simulink model "Fig264"  (R2014b)
settings: Solver=FixedStepDiscrete  StartTime=0.0  StopTime=.2  RelTol=1e-3
libraries: dspsigops x1
settings Model: Creator=Dennis Silage  LastModifiedBy=Silage
settings DataIOCC: SignalLoggingSaveFormat=ModelDataLogs
settings OptimizationCC: ExpressionDepthLimit=2147483647  InitFltsAndDblsToZero=on
settings DebuggingCC: UnderspecifiedInitializationDetection=Classic  MergeDetectMultiDrivingBlocksExec=none  FcnCallInpInsideContextMsg=UseLocalSettings  StateNameClashWarn=warning
settings GRTTargetCC: CombineOutputUpdateFcns=off  GRTInterface=on

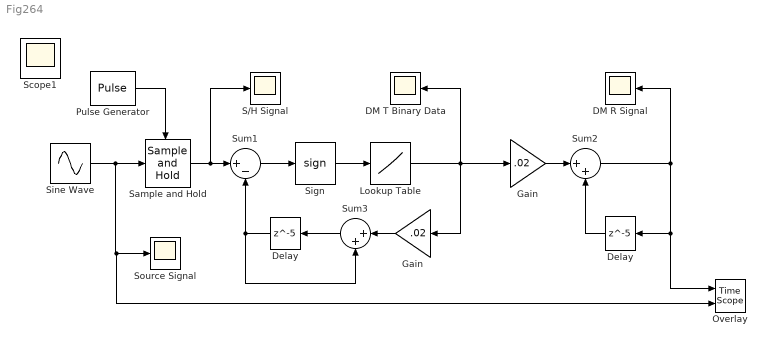
== system Fig264 ==
  DM R Signal : Scope
      settings: TimeRange=0.05  YMin=-8  YMax=8
  DM T Binary Data : Scope
      settings: TimeRange=0.05  YMin=-8  YMax=8
  Delay : Delay  DelayLength=5  InputProcessing=Inherited
  "Delay " : Delay  DelayLength=5  InputProcessing=Inherited
  Gain : Gain  Gain=.02
  "Gain " : Gain  Gain=.02
  Lookup Table : Lookup  InputValues=[-1,0,1]  Table=[-1,-1,1]
  Overlay : TimeScope  DefaultConfigurationName=spbscopes.TimeScopeBlockCfg  NumInputPorts=2
  Pulse Generator : DiscretePulseGenerator  PulseType=Time based  Period=5e-4  PulseWidth=20  VectorParams1D=off
  S/H Signal : Scope
      settings: TimeRange=0.05  YMin=-8  YMax=8  SaveName=ScopeData3
  Sample and Hold : dspsigops/Sample and Hold  trig=Rising edge  initCond=0  latchinput=off
  Sign : Signum
  Sine Wave : Sin  Frequency=20*pi  Samples=500000  SampleTime=1e-4  VectorParams1D=off
  Source Signal : Scope
      settings: TimeRange=0.05  YMin=-8  YMax=8  SaveName=ScopeData2
  Sum1 : Sum  Inputs=|+-
  Sum2 : Sum  Inputs=|++
  Sum3 : Sum  Inputs=|++
  Scope1 : Scope
      settings: YMin=-1.5  YMax=1.5  MaxDataPoints=7500  SampleTime=-1
  wires:
  Sum1/1 -> Sign/1
  Sine Wave/1 -> Sample and Hold/1, Overlay/2, Source Signal/1
  Sum3/1 -> Delay/1
  Sum2/1 -> Overlay/1, "Delay "/1, DM R Signal/1
  Delay/1 -> Sum1/2, Sum3/2
  "Delay "/1 -> Sum2/2
  Sample and Hold/1 -> Sum1/1, S/H Signal/1
  "Gain "/1 -> Sum2/1
  Sign/1 -> Lookup Table/1
  Gain/1 -> Sum3/1
  Lookup Table/1 -> "Gain "/1, DM T Binary Data/1, Gain/1
  Pulse Generator/1 -> Sample and Hold/Trigger
